simulink model "HVDC_breaker"  (R2020a)
settings: Solver=VariableStepAuto  StartTime=0.0  StopTime=2  RelTol=1e-3
libraries: powerlib x48, simulink_extras x2
settings Model: Creator=nitbh  LastModifiedBy=nitbh

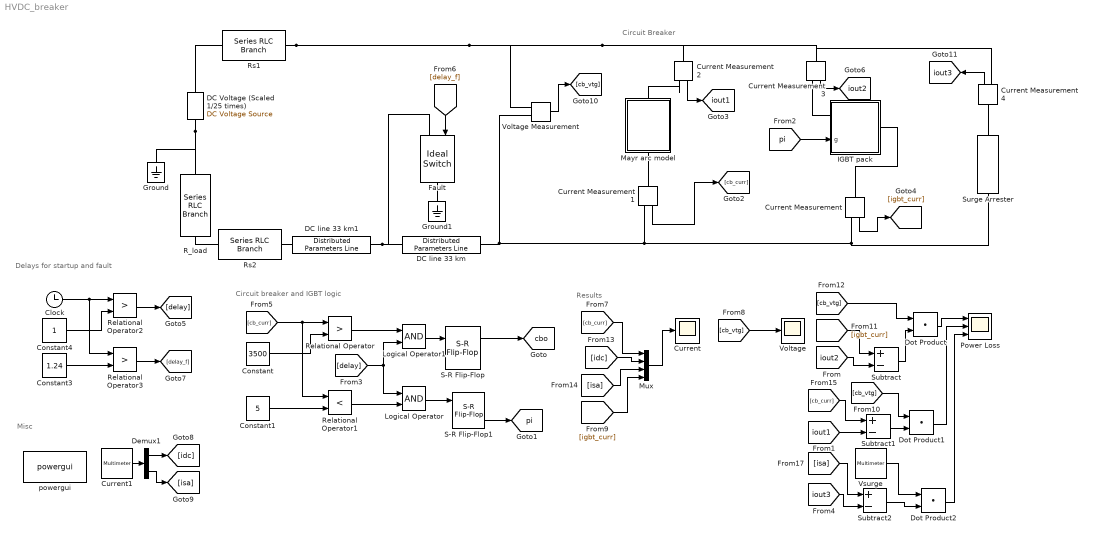
== system HVDC_breaker ==
  note: Delays for startup and fault
  note: Circuit breaker and IGBT logic
  note: Results
  note: Misc
  note: Circuit Breaker
  Clock : Clock
  Constant : Constant  Value=3500
  Constant1 : Constant  Value=5
  Constant3 : Constant  Value=1.24
  Constant4 : Constant
  Current : Scope
  Current Measurement{,1..4} (5 alike) : powerlib/Measurements/Current Measurement  PhasorSimulation=off  OutputType=Complex  PSBequivalent=0
  Current1 : powerlib/Measurements/Multimeter  PhasorSimulation=off  OutputType=Complex  sel=[12 14]  L=14  Gain=[1 1]  yselected={'Ib: Rs1','Ib: Surge Arrester'};  PSBOutputType=1  PSBequivalent=0  AxesSetting=[0,0.1,-100,100]  Display=0  SavedBlockNames=-11
  DC Voltage (Scaled 1/25 times) : powerlib/Electrical Sources/DC Voltage Source  Amplitude=20e3  Measurements=None
  DC line 33 km : powerlib/Elements/Distributed Parameters Line  Phases=1  Length=33  Frequency=60  Resistance=0.015  Inductance=0.792e-3  Capacitance=14.4e-9  x1=[1.12079363145529e-05;0;3.14159265822638]  x2=[1.18610734272342e-05;0;3.14159265781913]  x3=[1.36579236983347e-06;0;3.14159265108905]  x4=[1.26758136075432e-06;0;-3.03751646058004e-09]  x5=0.000111444278453405  V1=[1.121e-05;0;3.142]  V2=[1.186e-05;0;3.142]  I1=[1.366e-06;0;3.142]  I2=[1.268e-06;0;-3.038e-09]  nHarmo=1  Measurements=Phase-to-ground voltages  Decoupling=off  VsMag0=0  VrMag0=0  VsAngle0=0  VrAngle0=0  IsMag0=0  IrMag0=0  IsAngle0=0  IrAngle0=0
      settings: AttributesFormatString=\n
  DC line 33 km1 : powerlib/Elements/Distributed Parameters Line  Phases=1  Length=33  Frequency=60  Resistance=0.015  Inductance=0.792e-3  Capacitance=14.4e-9  x1=[1.05548546811563e-05;0;3.14159265868402]  x2=[1.12079363145529e-05;0;3.14159265822638]  x3=[1.36290006367565e-06;0;3.14159265108899]  x4=[1.27024998081597e-06;0;-3.03758351805072e-09]  x5=0.000111444278453405  V1=[1.055e-05;0;3.142]  V2=[1.121e-05;0;3.142]  I1=[1.363e-06;0;3.142]  I2=[1.27e-06;0;-3.038e-09]  nHarmo=1  Measurements=Phase-to-ground voltages  Decoupling=off  VsMag0=0  VrMag0=0  VsAngle0=0  VrAngle0=0  IsMag0=0  IrMag0=0  IsAngle0=0  IrAngle0=0
      settings: AttributesFormatString=\n
  Demux1 : Demux  Outputs=2
  Dot Product : DotProduct  InputSameDT=on  OutDataTypeStr=Inherit: Inherit via internal rule
  Dot Product1 : DotProduct  InputSameDT=on  OutDataTypeStr=Inherit: Inherit via internal rule
  Dot Product2 : DotProduct  InputSameDT=on  OutDataTypeStr=Inherit: Inherit via internal rule
  Fault : powerlib/Power Electronics/Ideal Switch  Ron=1e-7  Lon=0  IC=0  Rs=1e5  Cs=inf  Measurements=off
  Ground : powerlib/Elements/Ground  LConnTagsString=a
  Ground1 : powerlib/Elements/Ground  LConnTagsString=a
  IGBT pack : Subsystem
      settings: PortSchema="{\"entries\":[{\"content\":{\"sides\":[{\"content\":{\"connectorIds\":[\"LConn1\",\"In1\"]},\"type\":\"ConnectorPlacement.EquallySpacedRectSide\",\"uuid\":\"96d31f0d-7aa4-4057-b10d-93129c3218b2\"},{\"content\":{\"connectorIds\":[\"RConn1\"],\"side\":\"RIGHT\"},\"type\":\"ConnectorPlacement.EquallySpacedRectSide\",\"uuid\":\"db6d9455-2d8f-4413-b744-a87e6d3d38cd\"},{\"content\":{\"connectorIds\":[],\"side\":\"TOP\"},\"type\":\"ConnectorPlacement.EquallySpacedRectSide\",\"uuid\":\"40428968-9723-4ed6-afb8-e80947041635\"},{\"content\":{\"connectorIds\":[],\"side\":\"BOTTOM\"},\"type\":\"ConnectorPlacement.EquallySpacedRectSide\",\"uuid\":\"3bc59666-c7d8-490e-8b11-dc744ad3d8fc\"}]},\"type\":\"ConnectorPlacement.EquallySpacedConnector\",\"uuid\":\"f459b199-4a20-4f3f-a213-4896e45a2e8c\"}],\"packageUris\":[\"http://schema.mathworks.com/mf0/Connector/19700101\"],\"version\":\"1.0\"}"
  Logical Operator : Logic  AllPortsSameDT=off  OutDataTypeStr=boolean
  Logical Operator1 : Logic  AllPortsSameDT=off  OutDataTypeStr=boolean
  Mayr arc model : Subsystem  mask(Mayr arc model){tau=1e-4, P=30900e1, x0=1.e4, cb_trip=1.244, BAL=on, TC=1e-9}
      mask prompts: tau "tau [s]"; P "P [W]"; x0 "g(0) [S]"; cb_trip "circuit breaker contact separation starts at [s]"; BAL "Break algebraic loop"; TC "Time constant (Break algebraic loop in model)"
      mask help: The Mayr arc model with a constant time parameter tau and constant cooling power P: dlng/dt=1/tau*((ui/P)-1).
      mask init:
      | ME = get_param(gcb,'MaskEnables');
      | if BAL
      |     ME{end} = 'on';
      | else
      |     ME{end} = 'off';
      | end
      | set_param(gcb,'MaskEnables',ME);
      mask Help:
      | The Mayr arc model with a constant time parameter tau and constant cooling power P: dlng/dt=1/tau*((ui/P)-1).
      | 
      | The initial conductance of the arc g(0) can be altered. Furthermore, the time at which the contact separation of the circuit breaker takes place can be specified. Until that time the arc model behaves as a conductance with the value g(0).
      mask Display: plot(-15,10,115,90,[-15,15],[50,50],[85,115],[50,50],[15,15,25,25,15],[55,45,45,55,55],[75,75,85,85,75],[55,45,45,55,55],[25,75],[50,70])
  Mux : Mux
  Power Loss : Scope  NumInputPorts=3
  R_load : powerlib/Elements/Series RLC Branch  LConnTagsString=__new0  RConnTagsString=__new0  BranchType=R  Resistance=7  Inductance=0.1  SetiL0=on  InitialCurrent=2000  Capacitance=1e-6  Setx0=off  InitialVoltage=0  Measurements=Branch voltage and current
  Relational Operator : RelationalOperator  Operator=>  OutDataTypeStr=boolean  RndMeth=Simplest
  Relational Operator1 : RelationalOperator  Operator=<  OutDataTypeStr=boolean  RndMeth=Simplest
  Relational Operator2 : RelationalOperator  Operator=>  OutDataTypeStr=boolean  RndMeth=Simplest
  Relational Operator3 : RelationalOperator  Operator=>  OutDataTypeStr=boolean  RndMeth=Simplest
  Rs1 : powerlib/Elements/Series RLC Branch  LConnTagsString=__new0  RConnTagsString=__new0  BranchType=RL  Resistance=1  Inductance=0.02  SetiL0=on  InitialCurrent=2000  Capacitance=1e-6  Setx0=off  InitialVoltage=0  Measurements=Branch voltage and current
  Rs2 : powerlib/Elements/Series RLC Branch  LConnTagsString=__new0  RConnTagsString=__new0  BranchType=RL  Resistance=1  Inductance=0.001  SetiL0=on  InitialCurrent=2000  Capacitance=1e-6  Setx0=off  InitialVoltage=0  Measurements=Branch voltage and current
  S-R Flip-Flop : simulink_extras/Flip Flops/S-R Flip-Flop  initial_condition=0
  S-R Flip-Flop1 : simulink_extras/Flip Flops/S-R Flip-Flop  initial_condition=0
  Subtract : Sum  Inputs=+-
  Subtract1 : Sum  Inputs=+-
  Subtract2 : Sum  Inputs=+-
  Surge Arrester : powerlib/Elements/Surge Arrester  ProtectionVoltage=22.5e3  Columns=8  ReferenceCurrent=500  Segment1=[.955 50]  Segment2=[1.0 25]  Segment3=[.9915 16.5]  Measurements=Branch voltage and current  BreakLoop=off  UseDiscreteRobustSolver=on
      settings: SourceProductBaseCode=PS
  Voltage : Scope
  Voltage Measurement : powerlib/Measurements/Voltage Measurement  PhasorSimulation=off  OutputType=Complex  PSBequivalent=0
  Vsurge : powerlib/Measurements/Multimeter  PhasorSimulation=off  OutputType=Complex  sel=5  L=14  Gain=1  yselected={'Ub: Surge Arrester'};  PSBOutputType=1  PSBequivalent=0  AxesSetting=[0,0.1,-100,100]  Display=0  SavedBlockNames=-11
  powergui : powerlib/powergui  Priority=1  SimulationMode=Continuous  SampleTime=1e-5  frequency=60  Iterations=50  frequencyindice=0  Pbase=100e6  ErrMax=1e-4  UnitsV=kV  UnitsW=MW  buscounter=0  FunctionMessages=off  echomessages=off  EnableUseOfTLC=off  CurrentSourceSwitches=off  DisableSnubberDevices=off  DisableRonSwitches=off  DisableVfSwitches=off  DisplayEquations=off  AutomaticDiscreteSolvers=off  SolverType=Tustin/Backward Euler (TBE)  Interpol=off  ExternalGateDelay=off  methode=off  Ts=100  x0status=blocks  SPID=on  SwTol=0  HookPort=off  NonlinearTolerance=1e-4  nMaxIteration=100  ContinueOnMaxIteration=off  RestoreLinks=warning  ResistiveCurrentMeasurement=off  Frange=[0:2:500]  Ylog=off  Xlog=on  ShowGrid=off  save=off  variable=ZData  structure=0  ZoomFFT=off  StartTime=0.0  cycles=1  DisplayStyle=1  fundamental=60  FreqAxis=off  MaxFrequency=1000  frequencyindicesteady=1  RmsSteady=1  display=off
  tag scope: cbo=global, iout1=global, iout2=global, iout3=global, pi=global
  wires:
  [delay] -> Logical Operator1/2, Logical Operator/1
  Demux1/2 -> [isa]
  Logical Operator1/1 -> S-R Flip-Flop/1
  Current1/1 -> Demux1/1
  [igbt_curr] -> Subtract/1
  Current Measurement1/1 -> [cb_curr]
  Relational Operator1/1 -> Logical Operator/2
  Mux/1 -> Current/1
  Constant3/1 -> Relational Operator3/2
  [delay_f] -> Fault/1
  Constant4/1 -> Relational Operator2/2
  Constant/1 -> Relational Operator/2
  Current Measurement/1 -> [igbt_curr]
  [cb_curr] -> Relational Operator/1, Relational Operator1/1
  Constant1/1 -> Relational Operator1/2
  [idc] -> Mux/2
  [isa] -> Mux/3
  Dot Product2/1 -> Power Loss/3
  Demux1/1 -> [idc]
  [cb_vtg] -> Dot Product1/1
  Dot Product/1 -> Power Loss/1
  [cb_vtg] -> Dot Product/1
  Relational Operator3/1 -> [delay_f]
  Logical Operator/1 -> S-R Flip-Flop1/1
  Clock/1 -> Relational Operator2/1, Relational Operator3/1
  [cb_curr] -> Mux/1
  Relational Operator/1 -> Logical Operator1/1
  Dot Product1/1 -> Power Loss/2
  Vsurge/1 -> Dot Product2/1
  [cb_vtg] -> Voltage/1
  Relational Operator2/1 -> [delay]
  [igbt_curr] -> Mux/4
  Voltage Measurement/1 -> [cb_vtg]
  S-R Flip-Flop1/2 -> [pi]
  S-R Flip-Flop/1 -> [cbo]
  [pi] -> IGBT pack/1(g)
  [iout2] -> Subtract/2
  Subtract/1 -> Dot Product/2
  Subtract1/1 -> Dot Product1/2
  [iout1] -> Subtract1/2
  [cb_curr] -> Subtract1/1
  [isa] -> Subtract2/1
  [iout3] -> Subtract2/2
  Subtract2/1 -> Dot Product2/2
  Current Measurement2/1 -> [iout1]
  Current Measurement3/1 -> [iout2]
  Current Measurement4/1 -> [iout3]
  connections:
  DC line 33 km1/RConn1 -- Fault/LConn1 -- DC line 33 km/LConn1
  DC Voltage (Scaled 1/25 times)/LConn1 -- R_load/LConn1 -- Ground/LConn1
  Voltage Measurement/LConn2 -- DC line 33 km/RConn1 -- Surge Arrester/RConn1 -- Current Measurement/RConn1 -- Current Measurement1/RConn1
  Current Measurement1/LConn1 -- Mayr arc model/RConn1
  DC line 33 km1/LConn1 -- Rs2/RConn1
  Ground1/LConn1 -- Fault/RConn1
  Rs2/LConn1 -- R_load/RConn1
  DC Voltage (Scaled 1/25 times)/RConn1 -- Rs1/LConn1
  Rs1/RConn1 -- Voltage Measurement/LConn1 -- Current Measurement4/RConn1 -- Current Measurement3/LConn1 -- Current Measurement2/LConn1
  IGBT pack/RConn1 -- Current Measurement/LConn1
  Current Measurement2/RConn1 -- Mayr arc model/LConn1
  Current Measurement3/RConn1 -- IGBT pack/LConn1
  Current Measurement4/LConn1 -- Surge Arrester/LConn1

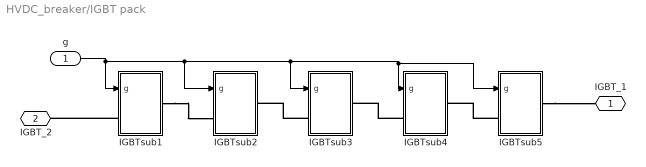
== system HVDC_breaker/IGBT pack ==
  g : Inport
  IGBTsub1 : Subsystem
  IGBTsub2 : Subsystem
  IGBTsub3 : Subsystem
  IGBTsub4 : Subsystem
  IGBTsub5 : Subsystem
  IGBT_1 : PMIOPort  Side=Left
  IGBT_2 : PMIOPort  Port=2  Side=Right
  wires:
  g/1 -> IGBTsub5/1(g), IGBTsub4/1(g), IGBTsub3/1(g), IGBTsub2/1(g), IGBTsub1/1(g)
  connections:
  IGBTsub1/LConn1 -- IGBT_2/RConn1
  IGBTsub5/RConn1 -- IGBT_1/RConn1
  IGBTsub4/LConn1 -- IGBTsub3/RConn1
  IGBTsub3/LConn1 -- IGBTsub2/RConn1
  IGBTsub1/RConn1 -- IGBTsub2/LConn1
  IGBTsub5/LConn1 -- IGBTsub4/RConn1

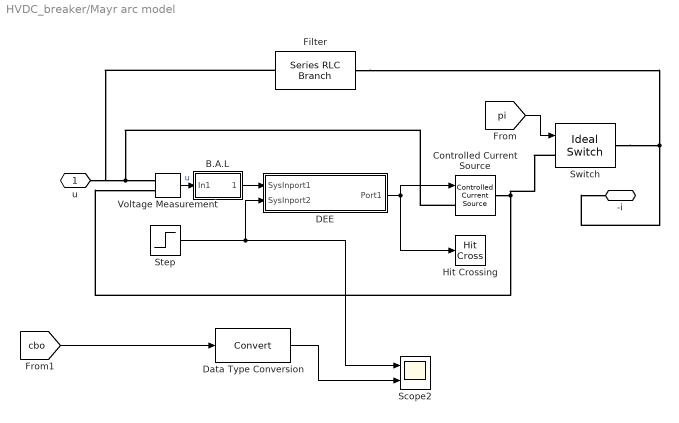
== system HVDC_breaker/Mayr arc model ==
  B.A.L : Subsystem
  Controlled Current Source : powerlib/Electrical Sources/Controlled Current Source  Description=source block  Initialize=on  Source_Type=AC  Amplitude=0  Phase=0  Frequency=0  Measurements=None
      settings: AttributesFormatString=\n
  DEE : Subsystem  mask(Differential Equation Editor (DEE)){}
      settings: OpenFcn=diffeqed
      mask Display: disp('Mayr arc model')
  Data Type Conversion : DataTypeConversion
  Filter : powerlib/Elements/Series RLC Branch  LConnTagsString=__new0  RConnTagsString=__new0  BranchType=C  Resistance=1  Inductance=0.01  SetiL0=on  InitialCurrent=2000  Capacitance=1e-6  Setx0=off  InitialVoltage=4e3  Measurements=Branch voltage and current
  Hit Crossing : HitCross  ZeroCross=off  ShowOutputPort=off
  Scope2 : Scope  NumInputPorts=2
  Step : Step  Time=cb_trip  SampleTime=0  ZeroCross=off
  Switch : powerlib/Power Electronics/Ideal Switch  Ron=1e-6  Lon=0  IC=1  Rs=1e5  Cs=inf  Measurements=off
  Voltage Measurement : powerlib/Measurements/Voltage Measurement  Tag=PoWeRsYsTeMmEaSuReMeNt  PhasorSimulation=off  OutputType=Magnitude  PSBequivalent=0
  u : PMIOPort  Side=Left
  -i : PMIOPort  Port=2  Side=Right
  wires:
  Step/1 -> Scope2/1, DEE/2(SysInport2)
  DEE/1(Port1) -> Hit Crossing/1, Controlled Current Source/1
  Voltage Measurement/1 -> B.A.L/1(In1)  "u"
  B.A.L/1(Out1) -> DEE/1(SysInport1)
  [pi] -> Switch/1
  [cbo] -> Data Type Conversion/1
  Data Type Conversion/1 -> Scope2/2
  connections:
  Controlled Current Source/RConn1 -- Switch/LConn1 -- Voltage Measurement/LConn2
  Controlled Current Source/LConn1 -- Filter/RConn1 -- u/RConn1 -- Voltage Measurement/LConn1
  Switch/RConn1 -- Filter/LConn1 -- -i/RConn1

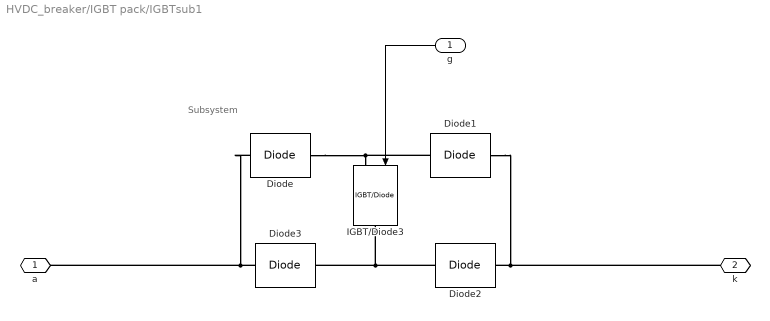
== system HVDC_breaker/IGBT pack/IGBTsub1 ==
  note: Subsystem
  g : Inport
  Diode : powerlib/Power Electronics/Diode  Ron=0.47e-3  Lon=0  Vf=2.3  IC=0  UseSnubber=0  Rs=500  Cs=250e-9  Measurements=off
  Diode1 : powerlib/Power Electronics/Diode  Ron=0.47e-3  Lon=0  Vf=2.3  IC=0  UseSnubber=0  Rs=500  Cs=250e-9  Measurements=off
  Diode2 : powerlib/Power Electronics/Diode  Ron=0.47e-3  Lon=0  Vf=2.3  IC=0  UseSnubber=0  Rs=500  Cs=250e-9  Measurements=off
  Diode3 : powerlib/Power Electronics/Diode  Ron=0.47e-3  Lon=0  Vf=0.8  IC=0  UseSnubber=0  Rs=500  Cs=250e-9  Measurements=off
  IGBT/Diode3 : powerlib/Power Electronics/IGBT//Diode  Ron=4e-4  Rs=1e2  Cs=1e-3  Measurements=off
  a : PMIOPort  Side=Left
  k : PMIOPort  Port=2  Side=Right
  wires:
  g/1 -> IGBT/Diode3/1
  connections:
  Diode1/LConn1 -- k/RConn1 -- Diode2/RConn1
  Diode2/LConn1 -- IGBT/Diode3/RConn1 -- Diode3/LConn1
  Diode3/RConn1 -- a/RConn1 -- Diode/LConn1
  Diode/RConn1 -- Diode1/RConn1 -- IGBT/Diode3/LConn1

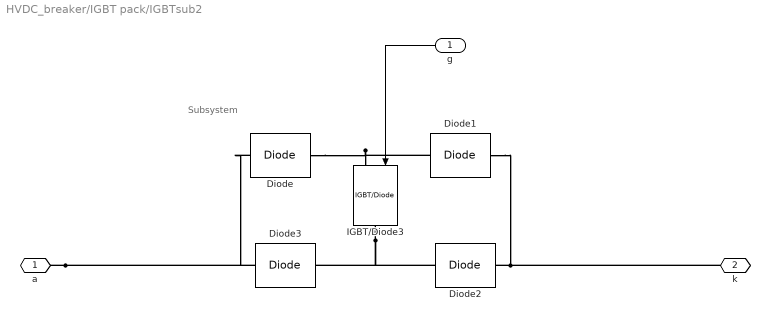
== system HVDC_breaker/IGBT pack/IGBTsub2 ==
  note: Subsystem
  g : Inport
  Diode : powerlib/Power Electronics/Diode  Ron=0.47e-3  Lon=0  Vf=2.3  IC=0  UseSnubber=0  Rs=500  Cs=250e-9  Measurements=off
  Diode1 : powerlib/Power Electronics/Diode  Ron=0.47e-3  Lon=0  Vf=2.3  IC=0  UseSnubber=0  Rs=500  Cs=250e-9  Measurements=off
  Diode2 : powerlib/Power Electronics/Diode  Ron=0.47e-3  Lon=0  Vf=2.3  IC=0  UseSnubber=0  Rs=500  Cs=250e-9  Measurements=off
  Diode3 : powerlib/Power Electronics/Diode  Ron=0.47e-3  Lon=0  Vf=0.8  IC=0  UseSnubber=0  Rs=500  Cs=250e-9  Measurements=off
  IGBT/Diode3 : powerlib/Power Electronics/IGBT//Diode  Ron=4e-4  Rs=1e2  Cs=1e-3  Measurements=off
  a : PMIOPort  Side=Left
  k : PMIOPort  Port=2  Side=Right
  wires:
  g/1 -> IGBT/Diode3/1
  connections:
  IGBT/Diode3/LConn1 -- Diode/RConn1 -- Diode1/RConn1
  a/RConn1 -- Diode/LConn1 -- Diode3/RConn1
  IGBT/Diode3/RConn1 -- Diode3/LConn1 -- Diode2/LConn1
  k/RConn1 -- Diode1/LConn1 -- Diode2/RConn1

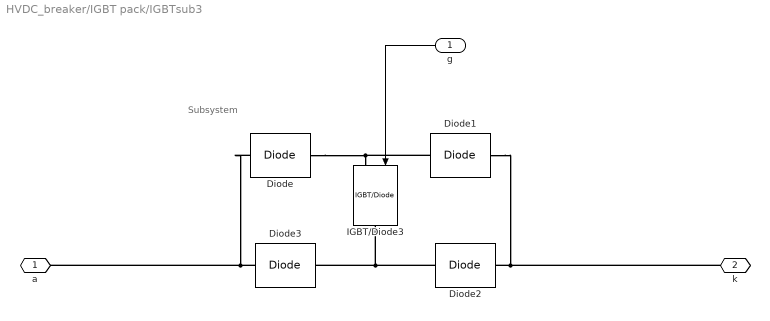
== system HVDC_breaker/IGBT pack/IGBTsub3 ==
  note: Subsystem
  g : Inport
  Diode : powerlib/Power Electronics/Diode  Ron=0.47e-3  Lon=0  Vf=2.3  IC=0  UseSnubber=0  Rs=500  Cs=250e-9  Measurements=off
  Diode1 : powerlib/Power Electronics/Diode  Ron=0.47e-3  Lon=0  Vf=2.3  IC=0  UseSnubber=0  Rs=500  Cs=250e-9  Measurements=off
  Diode2 : powerlib/Power Electronics/Diode  Ron=0.47e-3  Lon=0  Vf=2.3  IC=0  UseSnubber=0  Rs=500  Cs=250e-9  Measurements=off
  Diode3 : powerlib/Power Electronics/Diode  Ron=0.47e-3  Lon=0  Vf=0.8  IC=0  UseSnubber=0  Rs=500  Cs=250e-9  Measurements=off
  IGBT/Diode3 : powerlib/Power Electronics/IGBT//Diode  Ron=4e-4  Rs=1e2  Cs=1e-3  Measurements=off
  a : PMIOPort  Side=Left
  k : PMIOPort  Port=2  Side=Right
  wires:
  g/1 -> IGBT/Diode3/1
  connections:
  Diode2/RConn1 -- Diode1/LConn1 -- k/RConn1
  Diode2/LConn1 -- Diode3/LConn1 -- IGBT/Diode3/RConn1
  Diode3/RConn1 -- Diode/LConn1 -- a/RConn1
  Diode1/RConn1 -- Diode/RConn1 -- IGBT/Diode3/LConn1

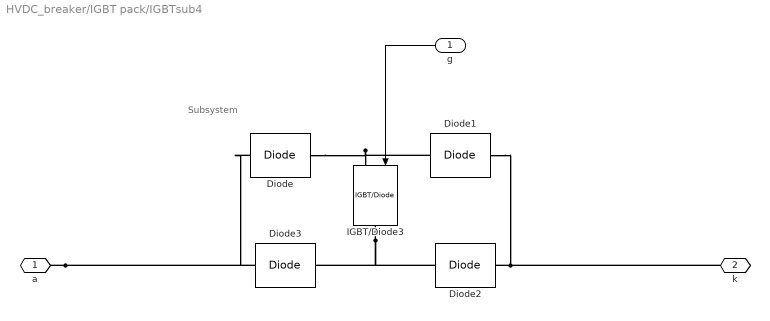
== system HVDC_breaker/IGBT pack/IGBTsub4 ==
  note: Subsystem
  g : Inport
  Diode : powerlib/Power Electronics/Diode  Ron=0.47e-3  Lon=0  Vf=2.3  IC=0  UseSnubber=0  Rs=500  Cs=250e-9  Measurements=off
  Diode1 : powerlib/Power Electronics/Diode  Ron=0.47e-3  Lon=0  Vf=2.3  IC=0  UseSnubber=0  Rs=500  Cs=250e-9  Measurements=off
  Diode2 : powerlib/Power Electronics/Diode  Ron=0.47e-3  Lon=0  Vf=2.3  IC=0  UseSnubber=0  Rs=500  Cs=250e-9  Measurements=off
  Diode3 : powerlib/Power Electronics/Diode  Ron=0.47e-3  Lon=0  Vf=0.8  IC=0  UseSnubber=0  Rs=500  Cs=250e-9  Measurements=off
  IGBT/Diode3 : powerlib/Power Electronics/IGBT//Diode  Ron=4e-4  Rs=1e2  Cs=1e-3  Measurements=off
  a : PMIOPort  Side=Left
  k : PMIOPort  Port=2  Side=Right
  wires:
  g/1 -> IGBT/Diode3/1
  connections:
  IGBT/Diode3/LConn1 -- Diode/RConn1 -- Diode1/RConn1
  a/RConn1 -- Diode/LConn1 -- Diode3/RConn1
  IGBT/Diode3/RConn1 -- Diode3/LConn1 -- Diode2/LConn1
  k/RConn1 -- Diode1/LConn1 -- Diode2/RConn1

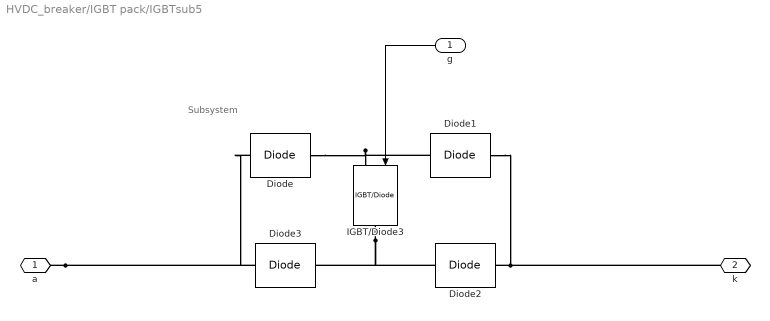
== system HVDC_breaker/IGBT pack/IGBTsub5 ==
  note: Subsystem
  g : Inport
  Diode : powerlib/Power Electronics/Diode  Ron=0.47e-3  Lon=0  Vf=2.3  IC=0  UseSnubber=0  Rs=500  Cs=250e-9  Measurements=off
  Diode1 : powerlib/Power Electronics/Diode  Ron=0.47e-3  Lon=0  Vf=2.3  IC=0  UseSnubber=0  Rs=500  Cs=250e-9  Measurements=off
  Diode2 : powerlib/Power Electronics/Diode  Ron=0.47e-3  Lon=0  Vf=2.3  IC=0  UseSnubber=0  Rs=500  Cs=250e-9  Measurements=off
  Diode3 : powerlib/Power Electronics/Diode  Ron=0.47e-3  Lon=0  Vf=0.8  IC=0  UseSnubber=0  Rs=500  Cs=250e-9  Measurements=off
  IGBT/Diode3 : powerlib/Power Electronics/IGBT//Diode  Ron=4e-4  Rs=1e2  Cs=1e-3  Measurements=off
  a : PMIOPort  Side=Left
  k : PMIOPort  Port=2  Side=Right
  wires:
  g/1 -> IGBT/Diode3/1
  connections:
  IGBT/Diode3/LConn1 -- Diode/RConn1 -- Diode1/RConn1
  a/RConn1 -- Diode/LConn1 -- Diode3/RConn1
  IGBT/Diode3/RConn1 -- Diode3/LConn1 -- Diode2/LConn1
  k/RConn1 -- Diode1/LConn1 -- Diode2/RConn1

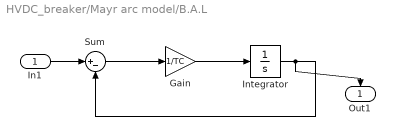
== system HVDC_breaker/Mayr arc model/B.A.L ==
  In1 : Inport
  Gain : Gain  Gain=1/TC
  Integrator : Integrator
  Sum : Sum  Inputs=|+-
  Out1 : Outport  InitialOutput=0  VectorParamsAs1DForOutWhenUnconnected=off
  wires:
  Gain/1 -> Integrator/1
  Integrator/1 -> Sum/2, Out1/1
  Sum/1 -> Gain/1
  In1/1 -> Sum/1

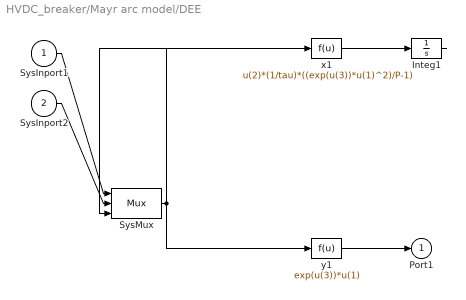
== system HVDC_breaker/Mayr arc model/DEE ==
  SysInport1 : Inport
  SysInport2 : Inport  Port=2
  Integ1 : Integrator  InitialCondition=log(x0)  ZeroCross=off
  SysMux : Mux  Inputs=3
  x1 : Fcn  Expr=u(2)*(1/tau)*((exp(u(3))*u(1)^2)/P-1)
  y1 : Fcn  Expr=exp(u(3))*u(1)
  Port1 : Outport  InitialOutput=0  VectorParamsAs1DForOutWhenUnconnected=off
  wires:
  y1/1 -> Port1/1
  SysMux/1 -> y1/1, x1/1
  Integ1/1 -> SysMux/3
  x1/1 -> Integ1/1
  SysInport2/1 -> SysMux/2
  SysInport1/1 -> SysMux/1
